simulink model "r_controller_system_integrated"  (R2025b)
settings: Solver=ode5  StartTime=0.0  StopTime=0.1  FixedStep=1e-05  MaxStep=1e-06  RelTol=1e-3
values from neighbouring files (symbols this model uses):
  params = Simulink.Parameter(params_data)    [r_controller_calc_params.m]
undefined symbols (not defined in the file or in its folder): Amplitude, Channel, ControllerType, d, Frequency, Ki_value, Kp_value, Phase, SignalType, StepTime
libraries: slpidlib x6, simulink x1
settings Model: Creator=PME406_01  LastModifiedBy=PME406_01
settings DebuggingCC: MergeDetectMultiDrivingBlocksExec=none
settings ModelReferenceCC: PropagateSignalLabelsOutOfModel=off

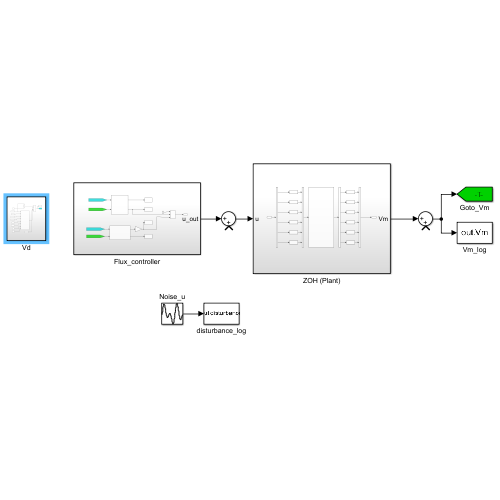
[thumbnail: Simulink's stored preview of the top-level diagram]
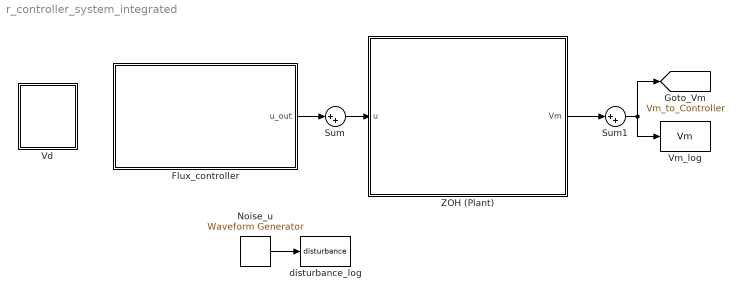
== system r_controller_system_integrated ==
  Flux_controller : Subsystem
  Noise_u : simulink/Sources/Waveform Generator  OutMin=[]  OutMax=[]  OutDataTypeStr=double  SelectedSignal=5  Signals=sin(0.1,10*2*pi, 0) + sin(0.1, 100*2*pi, pi/2) +sin(0.1,1000*2*pi, pi/4)#square(0.1,1000*2*pi,0,50)+square(0.1,500*2*pi,0,50)+square(0.1,50*2*pi,0,50)#sin(0.1,100*2*pi, pi/4)+sin(0.1,3000*2*pi,0)#square(0.1,50*2*pi,0,50)#sin(0.3, 100*2*pi, 0)#sawtooth(0.15,100*2*pi, pi/2)+sin(0.3, 100*2*pi, 0)#  BlockNames=MultiportSwitch_6f71199b286f490#MultiportSwitch_dade89289388493#MultiportSwitch_cf8a6d85c6a04a6#MultiportSwitch_8069dea399c144f#MultiportSwitch_735d7398da51477#MultiportSwitch_ae675588fc81459#MultiportSwitch_89d8400a71a24e9  SampleTime=1e-5
  Sum : Sum  Inputs=|++
  Sum1 : Sum  Inputs=|++
  Vd : Subsystem
  Vm_log : ToWorkspace  VariableName=Vm  SampleTime=1e-5
      settings: Save2DSignal=2-D array (concatenate along first dimension)
  ZOH (Plant) : Subsystem
  disturbance_log : ToWorkspace  VariableName=disturbance  SampleTime=1e-5
      settings: Save2DSignal=2-D array (concatenate along first dimension)
  tag scope: Vm_to_Controller=global
  wires:
  Noise_u/1 -> disturbance_log/1
  Sum1/1 -> Vm_log/1, [Vm_to_Controller]
  Sum/1 -> ZOH (Plant)/1(u)
  ZOH (Plant)/1(Vm) -> Sum1/1
  Flux_controller/1(u_out) -> Sum/1

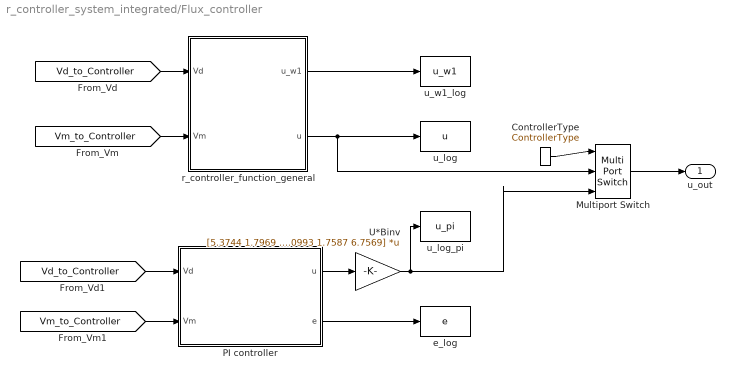
== system r_controller_system_integrated/Flux_controller ==
  ControllerType : Constant  Value=ControllerType
  Multiport Switch : MultiPortSwitch  Inputs=2  SaturateOnIntegerOverflow=off  InputSameDT=off
  PI controller : Subsystem
  U*Binv : Gain  Gain=[5.3744 1.7969 1.7574 2.2456 2.2738 2.0311;1.5722 5.8626 2.1621 3.1898 3.2303 2.3567;1.7622 2.0686 5.9804 1.8643 2.1053 2.1404;1.9445 3.4221 1.8713 6.8989 3.6309 2.3796;2.0590 3.2035 2.0193 3.4407 6.4464 2.0016;1.5291 2.0809 1.7335 2.0993 1.7587 6.7569]  Multiplication=Matrix(K*u)
  e_log : ToWorkspace  VariableName=e  SampleTime=-1
      settings: Save2DSignal=2-D array (concatenate along first dimension)
  r_controller_function_general : Subsystem
  u_log : ToWorkspace  VariableName=u  SampleTime=1e-5
      settings: Save2DSignal=2-D array (concatenate along first dimension)
  u_log_pi : ToWorkspace  VariableName=u_pi  SampleTime=-1
      settings: Save2DSignal=2-D array (concatenate along first dimension)
  u_w1_log : ToWorkspace  VariableName=u_w1  SampleTime=1e-5
      settings: Save2DSignal=2-D array (concatenate along first dimension)
  u_out : Outport
  wires:
  [Vd_to_Controller] -> r_controller_function_general/1(Vd)
  PI controller/1(u) -> U*Binv/1
  [Vd_to_Controller] -> PI controller/1(Vd)
  U*Binv/1 -> u_log_pi/1, Multiport Switch/3
  ControllerType/1 -> Multiport Switch/1
  [Vm_to_Controller] -> PI controller/2(Vm)
  r_controller_function_general/1(u_w1) -> u_w1_log/1
  r_controller_function_general/2(u) -> u_log/1, Multiport Switch/2
  [Vm_to_Controller] -> r_controller_function_general/2(Vm)
  PI controller/2(e) -> e_log/1
  Multiport Switch/1 -> u_out/1

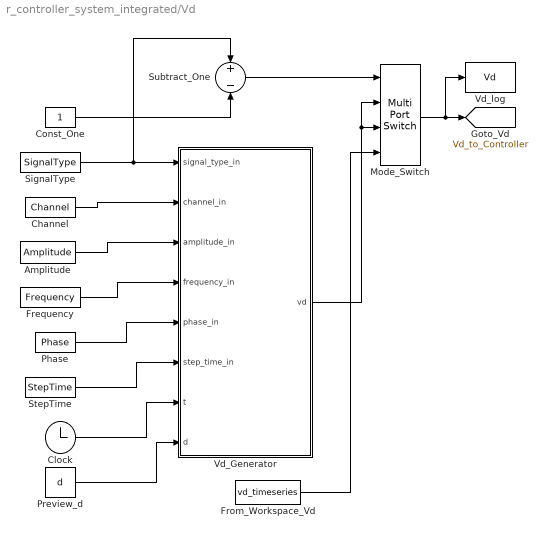
== system r_controller_system_integrated/Vd ==
  Amplitude : Constant  Value=Amplitude
  Channel : Constant  Value=Channel
  Clock : Clock
  Const_One : Constant
  Frequency : Constant  Value=Frequency
  From_Workspace_Vd : FromWorkspace  VariableName=vd_timeseries  SampleTime=1e-5  OutputAfterFinalValue=Holding final value
  Mode_Switch : MultiPortSwitch  DataPortOrder=Zero-based contiguous  zeroidx=on  SaturateOnIntegerOverflow=off  InputSameDT=off
  Phase : Constant  Value=Phase
  Preview_d : Constant  Value=d
  SignalType : Constant  Value=SignalType
  StepTime : Constant  Value=StepTime
  Subtract_One : Sum  Inputs=+-
  Vd_Generator : MATLAB Function  TreatAsAtomicUnit=on
  Vd_log : ToWorkspace  VariableName=Vd  SampleTime=1e-5
      settings: Save2DSignal=2-D array (concatenate along first dimension)
  tag scope: Vd_to_Controller=global
  wires:
  From_Workspace_Vd/1 -> Mode_Switch/4
  Vd_Generator/1(vd) -> Mode_Switch/3, Mode_Switch/2
  Preview_d/1 -> Vd_Generator/8(d)
  Clock/1 -> Vd_Generator/7(t)
  Frequency/1 -> Vd_Generator/4(frequency_in)
  StepTime/1 -> Vd_Generator/6(step_time_in)
  Channel/1 -> Vd_Generator/2(channel_in)
  Phase/1 -> Vd_Generator/5(phase_in)
  Amplitude/1 -> Vd_Generator/3(amplitude_in)
  Subtract_One/1 -> Mode_Switch/1
  SignalType/1 -> Vd_Generator/1(signal_type_in), Subtract_One/1
  Const_One/1 -> Subtract_One/2
  Mode_Switch/1 -> Vd_log/1, [Vd_to_Controller]

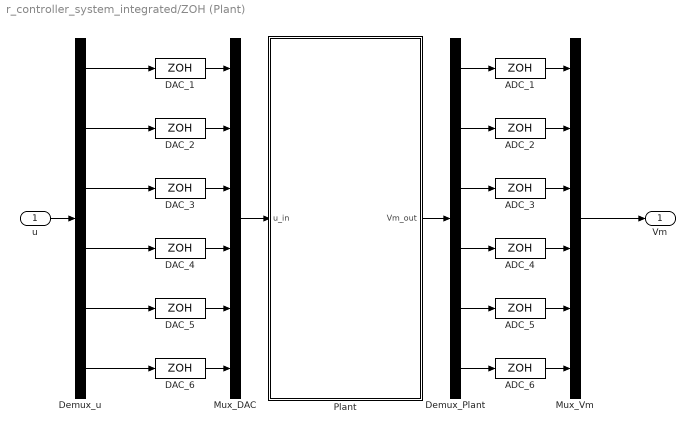
== system r_controller_system_integrated/ZOH (Plant) ==
  u : Inport
  ADC_{1..6} (6 alike) : ZeroOrderHold  SampleTime=1e-05
  DAC_{1..6} (6 alike) : ZeroOrderHold  SampleTime=1e-05
  Demux_Plant : Demux  Outputs=6
  Demux_u : Demux  Outputs=6
  Mux_DAC : Mux  Inputs=6
  Mux_Vm : Mux  Inputs=6
  Plant : Subsystem
  Vm : Outport
  wires:
  Demux_Plant/3 -> ADC_3/1
  DAC_2/1 -> Mux_DAC/2
  Demux_u/1 -> DAC_1/1
  Demux_u/6 -> DAC_6/1
  ADC_4/1 -> Mux_Vm/4
  DAC_3/1 -> Mux_DAC/3
  Mux_Vm/1 -> Vm/1
  Demux_Plant/2 -> ADC_2/1
  ADC_6/1 -> Mux_Vm/6
  Demux_Plant/1 -> ADC_1/1
  ADC_2/1 -> Mux_Vm/2
  Demux_u/5 -> DAC_5/1
  Plant/1(Vm_out) -> Demux_Plant/1
  Mux_DAC/1 -> Plant/1(u_in)
  DAC_1/1 -> Mux_DAC/1
  ADC_1/1 -> Mux_Vm/1
  Demux_u/4 -> DAC_4/1
  Demux_u/3 -> DAC_3/1
  Demux_Plant/6 -> ADC_6/1
  Demux_Plant/4 -> ADC_4/1
  ADC_3/1 -> Mux_Vm/3
  Demux_Plant/5 -> ADC_5/1
  DAC_4/1 -> Mux_DAC/4
  ADC_5/1 -> Mux_Vm/5
  DAC_5/1 -> Mux_DAC/5
  DAC_6/1 -> Mux_DAC/6
  Demux_u/2 -> DAC_2/1
  u/1 -> Demux_u/1

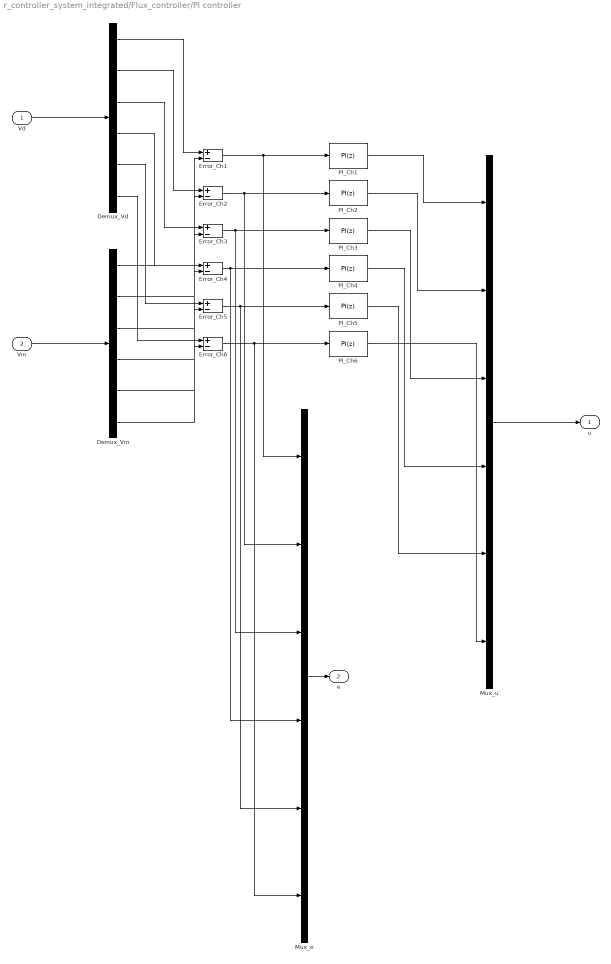
== system r_controller_system_integrated/Flux_controller/PI controller ==
  Vd : Inport
  Vm : Inport  Port=2
  Demux_Vd : Demux  Outputs=6
  Demux_Vm : Demux  Outputs=6
  Error_Ch{1..6} (6 alike) : Sum  Inputs=+-
  Mux_e : Mux  Inputs=6
  Mux_u : Mux  Inputs=6
  PI_Ch{1..2,4..6} (5 alike) : slpidlib/PID Controller  Controller=PI  Form=Parallel  TimeDomain=Discrete-time  UseExternalTs=off  SampleTime=1e-5  IntegratorMethod=Trapezoidal  FilterMethod=Forward Euler  ControllerParametersSource=internal  P=Kp_value  I=Ki_value  UseKiTs=off  D=0  UseExternalDerivativeSource=off  N=100  UseFilter=on  TunerSelectOption=Transfer Function Based (PID Tuner App)  InitialConditionSource=internal  InitialConditionForIntegrator=0  InitialConditionForFilter=0  DifferentiatorICPrevScaledInput=0  ExternalReset=none  TrackingMode=off  Kt=1  LimitOutput=off  SatLimitsSource=internal  UpperSaturationLimit=10  LowerSaturationLimit=-10  LinearizeAsGain=off  AntiWindupMode=back-calculation  Kb=1  LimitIntegrator=off  UpperIntegratorSaturationLimit=inf  LowerIntegratorSaturationLimit=-inf  POutMin=[]  POutMax=[]  IOutMin=[]  IOutMax=[]  DOutMin=[]  DOutMax=[]  NOutMin=[]  NOutMax=[]  SumOutMin=[]  SumOutMax=[]  SaturationOutMin=[]  SaturationOutMax=[]  PParamMin=[]  PParamMax=[]  IParamMin=[]  IParamMax=[]  DParamMin=[]  DParamMax=[]  NParamMin=[]  NParamMax=[]  KbParamMin=[]  KbParamMax=[]  KtParamMin=[]  KtParamMax=[]  KbOutMin=[]  KbOutMax=[]  KtOutMin=[]  KtOutMax=[]  IntegratorOutMin=[]  IntegratorOutMax=[]  FilterOutMin=[]  FilterOutMax=[]  SumI1OutMin=[]  SumI1OutMax=[]  SumI2OutMin=[]  SumI2OutMax=[]  SumI3OutMin=[]  SumI3OutMax=[]  SumI4OutMin=[]  SumI4OutMax=[]  SumDOutMin=[]  SumDOutMax=[]  DifferentiatorOutMin=[]  DifferentiatorOutMax=[]  FilterDiffOutCoefMin=[]  FilterDiffOutCoefMax=[]  ReciprocalOutMin=[]  ReciprocalOutMax=[]  SumDenOutMin=[]  SumDenOutMax=[]  SumNumOutMin=[]  SumNumOutMax=[]  DivideOutMin=[]  DivideOutMax=[]  UdiffTsProdOutMin=[]  UdiffTsProdOutMax=[]  NTsProdOutMin=[]  NTsProdOutMax=[]  UintegralTsProdOutMin=[]  UintegralTsProdOutMax=[]  UngainTsProdOutMin=[]  UngainTsProdOutMax=[]  ClampingZeroOutDataTypeStr=Inherit: Inherit via back propagation  ClampingZeroOutMin=[]  ClampingZeroOutMax=[]  FilterDenConstantOutDataTypeStr=Inherit: Inherit via back propagation  FilterDenConstantOutMin=[]  FilterDenConstantOutMax=[]  PCopyOutDataTypeStr=Inherit: Inherit via back propagation  PCopyOutMin=[]  PCopyOutMax=[]  NCopyOutDataTypeStr=Inherit: Inherit via back propagation  NCopyOutMin=[]  NCopyOutMax=[]  IntegratorContinuousStateAttributes=''  IntegratorStateMustResolveToSignalObject=off  IntegratorRTWStateStorageClass=Auto  FilterContinuousStateAttributes=''  FilterStateMustResolveToSignalObject=off  FilterRTWStateStorageClass=Auto  ParallelPVariant=InternalParameters  IdealPVariant=Disabled  IVariant=InternalParameters  DVariant=Disabled  IntegratorVariant=Discrete  SatVariant=Disabled  AWVariant=Passthrough  PCopyVariant=Disabled  TRVariant=Disabled  FdbkBlocksVariant=Forward  IdealPFdbkVariant=Disabled  SatFdbkVariant=Disabled  DerivativeFilterVariant=Disabled  NVariant=Disabled  NCopyVariant=Disabled_SignalSpec  FilterICVariant=Disabled  IntegratorICVariant=InternalICs  ExternalResetVariant=Disabled  TRSumVariant=Passthrough  SumFdbkVariant=Disabled  SumVariant=Sum_PI  TsampFilterVariant=InternalTs  TsampNgainVariant=Passthrough  TsampIntegralVariant=Disabled_SignalSpec  ExternalSaturationOutDataTypeStr=Inherit: Same as second input  DerivativeSourceVariant=Disabled  PreIntVariant=InternalPreInt
      settings: LibrarySourceBlock=simulink/Discrete/Discrete PID Controller
  PI_Ch3 : slpidlib/PID Controller  Controller=PI  Form=Parallel  TimeDomain=Discrete-time  UseExternalTs=off  SampleTime=1e-5  IntegratorMethod=Trapezoidal  FilterMethod=Forward Euler  ControllerParametersSource=internal  P=Kp_value  I=Ki_value  UseKiTs=off  D=0  UseExternalDerivativeSource=off  N=100  UseFilter=on  TunerSelectOption=Transfer Function Based (PID Tuner App)  InitialConditionSource=internal  InitialConditionForIntegrator=0  InitialConditionForFilter=0  DifferentiatorICPrevScaledInput=0  ExternalReset=none  TrackingMode=off  Kt=1  LimitOutput=off  SatLimitsSource=internal  UpperSaturationLimit=10  LowerSaturationLimit=-10  LinearizeAsGain=off  AntiWindupMode=back-calculation  Kb=1  LimitIntegrator=off  UpperIntegratorSaturationLimit=15  LowerIntegratorSaturationLimit=-15  POutMin=[]  POutMax=[]  IOutMin=[]  IOutMax=[]  DOutMin=[]  DOutMax=[]  NOutMin=[]  NOutMax=[]  SumOutMin=[]  SumOutMax=[]  SaturationOutMin=[]  SaturationOutMax=[]  PParamMin=[]  PParamMax=[]  IParamMin=[]  IParamMax=[]  DParamMin=[]  DParamMax=[]  NParamMin=[]  NParamMax=[]  KbParamMin=[]  KbParamMax=[]  KtParamMin=[]  KtParamMax=[]  KbOutMin=[]  KbOutMax=[]  KtOutMin=[]  KtOutMax=[]  IntegratorOutMin=[]  IntegratorOutMax=[]  FilterOutMin=[]  FilterOutMax=[]  SumI1OutMin=[]  SumI1OutMax=[]  SumI2OutMin=[]  SumI2OutMax=[]  SumI3OutMin=[]  SumI3OutMax=[]  SumI4OutMin=[]  SumI4OutMax=[]  SumDOutMin=[]  SumDOutMax=[]  DifferentiatorOutMin=[]  DifferentiatorOutMax=[]  FilterDiffOutCoefMin=[]  FilterDiffOutCoefMax=[]  ReciprocalOutMin=[]  ReciprocalOutMax=[]  SumDenOutMin=[]  SumDenOutMax=[]  SumNumOutMin=[]  SumNumOutMax=[]  DivideOutMin=[]  DivideOutMax=[]  UdiffTsProdOutMin=[]  UdiffTsProdOutMax=[]  NTsProdOutMin=[]  NTsProdOutMax=[]  UintegralTsProdOutMin=[]  UintegralTsProdOutMax=[]  UngainTsProdOutMin=[]  UngainTsProdOutMax=[]  ClampingZeroOutDataTypeStr=Inherit: Inherit via back propagation  ClampingZeroOutMin=[]  ClampingZeroOutMax=[]  FilterDenConstantOutDataTypeStr=Inherit: Inherit via back propagation  FilterDenConstantOutMin=[]  FilterDenConstantOutMax=[]  PCopyOutDataTypeStr=Inherit: Inherit via back propagation  PCopyOutMin=[]  PCopyOutMax=[]  NCopyOutDataTypeStr=Inherit: Inherit via back propagation  NCopyOutMin=[]  NCopyOutMax=[]  IntegratorContinuousStateAttributes=''  IntegratorStateMustResolveToSignalObject=off  IntegratorRTWStateStorageClass=Auto  FilterContinuousStateAttributes=''  FilterStateMustResolveToSignalObject=off  FilterRTWStateStorageClass=Auto  ParallelPVariant=InternalParameters  IdealPVariant=Disabled  IVariant=InternalParameters  DVariant=Disabled  IntegratorVariant=Discrete  SatVariant=Disabled  AWVariant=Passthrough  PCopyVariant=Disabled  TRVariant=Disabled  FdbkBlocksVariant=Forward  IdealPFdbkVariant=Disabled  SatFdbkVariant=Disabled  DerivativeFilterVariant=Disabled  NVariant=Disabled  NCopyVariant=Disabled_SignalSpec  FilterICVariant=Disabled  IntegratorICVariant=InternalICs  ExternalResetVariant=Disabled  TRSumVariant=Passthrough  SumFdbkVariant=Disabled  SumVariant=Sum_PI  TsampFilterVariant=InternalTs  TsampNgainVariant=Passthrough  TsampIntegralVariant=Disabled_SignalSpec  ExternalSaturationOutDataTypeStr=Inherit: Same as second input  DerivativeSourceVariant=Disabled  PreIntVariant=InternalPreInt
      settings: LibrarySourceBlock=simulink/Discrete/Discrete PID Controller
  u : Outport
  e : Outport  Port=2
  wires:
  Vd/1 -> Demux_Vd/1
  Vm/1 -> Demux_Vm/1
  Error_Ch5/1 -> PI_Ch5/1, Mux_e/5
  Demux_Vm/2 -> Error_Ch2/2
  Mux_u/1 -> u/1
  PI_Ch1/1 -> Mux_u/1
  PI_Ch4/1 -> Mux_u/4
  Error_Ch1/1 -> PI_Ch1/1, Mux_e/1
  Error_Ch3/1 -> PI_Ch3/1, Mux_e/3
  PI_Ch3/1 -> Mux_u/3
  Error_Ch6/1 -> PI_Ch6/1, Mux_e/6
  Error_Ch2/1 -> PI_Ch2/1, Mux_e/2
  Demux_Vm/5 -> Error_Ch5/2
  Demux_Vm/1 -> Error_Ch1/2
  Demux_Vd/2 -> Error_Ch2/1
  Demux_Vd/1 -> Error_Ch1/1
  PI_Ch2/1 -> Mux_u/2
  Demux_Vm/4 -> Error_Ch4/2
  Mux_e/1 -> e/1
  Demux_Vd/3 -> Error_Ch3/1
  Demux_Vd/6 -> Error_Ch6/1
  Error_Ch4/1 -> PI_Ch4/1, Mux_e/4
  Demux_Vd/5 -> Error_Ch5/1
  PI_Ch6/1 -> Mux_u/6
  PI_Ch5/1 -> Mux_u/5
  Demux_Vm/6 -> Error_Ch6/2
  Demux_Vm/3 -> Error_Ch3/2
  Demux_Vd/4 -> Error_Ch4/1

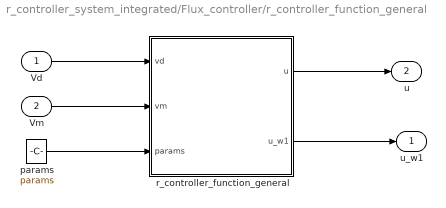
== system r_controller_system_integrated/Flux_controller/r_controller_function_general ==
  Vd : Inport
  Vm : Inport  Port=2
  params : Constant  Value=params  OutDataTypeStr=Bus: ParamsBus
  r_controller_function_general : MATLAB Function  TreatAsAtomicUnit=on
  u_w1 : Outport
  u : Outport  Port=2
  wires:
  r_controller_function_general/2(u_w1) -> u_w1/1
  Vm/1 -> r_controller_function_general/2(vm)
  Vd/1 -> r_controller_function_general/1(vd)
  r_controller_function_general/1(u) -> u/1
  params/1 -> r_controller_function_general/3(params)

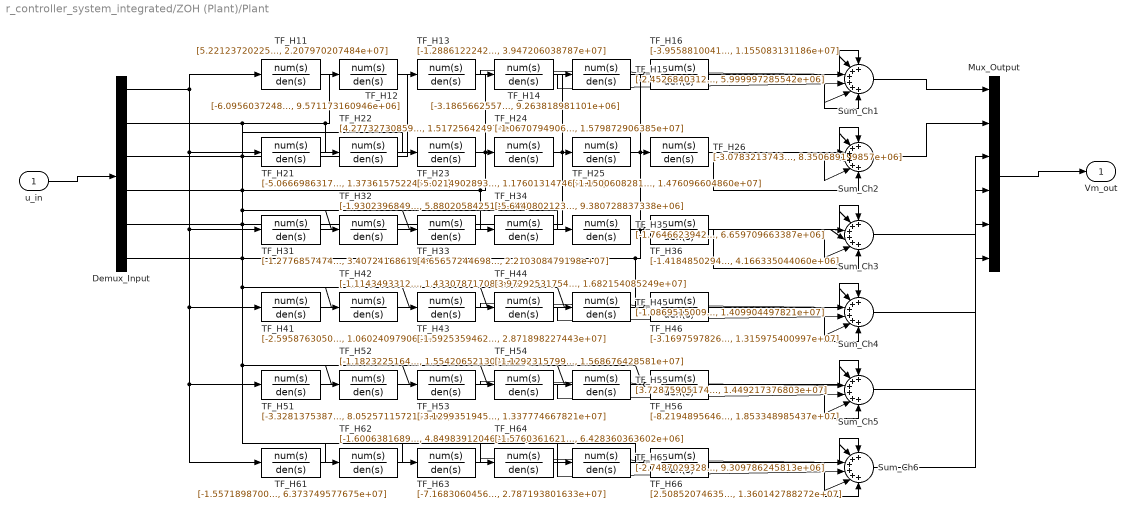
== system r_controller_system_integrated/ZOH (Plant)/Plant ==
  u_in : Inport
  Demux_Input : Demux  Outputs=6
  Mux_Output : Mux  Inputs=6
  Sum_Ch{1..6} (6 alike) : Sum  Inputs=++++++
  TF_H11 : TransferFcn  Numerator=[5.221237202258e+06]  Denominator=[1, 1.125476429798e+04, 2.207970207484e+07]
  TF_H12 : TransferFcn  Numerator=[-6.095603724823e+04]  Denominator=[1, 1.615096196557e+03, 9.571173160946e+06]
  TF_H13 : TransferFcn  Numerator=[-1.288612224236e+06]  Denominator=[1, 1.231137597589e+04, 3.947206038787e+07]
  TF_H14 : TransferFcn  Numerator=[-3.186566255776e+05]  Denominator=[1, 7.765927137710e+03, 9.263818981101e+06]
  TF_H15 : TransferFcn  Numerator=[-2.452684031253e+05]  Denominator=[1, 5.746401647961e+03, 5.999997285542e+06]
  TF_H16 : TransferFcn  Numerator=[-3.955881004140e+05]  Denominator=[1, 3.580306515557e+03, 1.155083131186e+07]
  TF_H21 : TransferFcn  Numerator=[-5.066698631790e+04]  Denominator=[1, 1.108261849372e+03, 1.373615752245e+07]
  TF_H22 : TransferFcn  Numerator=[4.277327308593e+06]  Denominator=[1, 1.003268373777e+04, 1.517256424974e+07]
  TF_H23 : TransferFcn  Numerator=[-5.021490289304e+05]  Denominator=[1, 8.810895080316e+03, 1.176013147465e+07]
  TF_H24 : TransferFcn  Numerator=[-1.067079490600e+06]  Denominator=[1, 1.135112820448e+04, 1.579872906385e+07]
  TF_H25 : TransferFcn  Numerator=[-1.150060828107e+06]  Denominator=[1, 1.065992916636e+04, 1.476096604860e+07]
  TF_H26 : TransferFcn  Numerator=[-3.078321374306e+05]  Denominator=[1, 6.847783968129e+03, 8.350689199857e+06]
  TF_H31 : TransferFcn  Numerator=[-1.277685747428e+06]  Denominator=[1, 1.368269686933e+04, 3.407241686199e+07]
  TF_H32 : TransferFcn  Numerator=[-1.930239684968e+05]  Denominator=[1, 4.560870597302e+03, 5.880205842512e+06]
  TF_H33 : TransferFcn  Numerator=[4.656572446985e+06]  Denominator=[1, 9.513164457161e+03, 2.210308479198e+07]
  TF_H34 : TransferFcn  Numerator=[-5.644080212304e+04]  Denominator=[1, 1.954878812118e+03, 9.380728837338e+06]
  TF_H35 : TransferFcn  Numerator=[-1.764662394212e+05]  Denominator=[1, 5.122349981324e+03, 6.659709663387e+06]
  TF_H36 : TransferFcn  Numerator=[-1.418485029440e+05]  Denominator=[1, 1.438504147902e+03, 4.166335044060e+06]
  TF_H41 : TransferFcn  Numerator=[-2.595876305066e+05]  Denominator=[1, 7.070165651413e+03, 1.060240979066e+07]
  TF_H42 : TransferFcn  Numerator=[-1.114349331223e+06]  Denominator=[1, 9.846928206402e+03, 1.433078717084e+07]
  TF_H43 : TransferFcn  Numerator=[-1.592535946272e+05]  Denominator=[1, 2.790294019501e+03, 2.871898227443e+07]
  TF_H44 : TransferFcn  Numerator=[3.972925317547e+06]  Denominator=[1, 1.159715140811e+04, 1.682154085249e+07]
  TF_H45 : TransferFcn  Numerator=[-1.086951500933e+06]  Denominator=[1, 1.075231371220e+04, 1.409904497821e+07]
  TF_H46 : TransferFcn  Numerator=[-3.169759782656e+05]  Denominator=[1, 8.067558736035e+03, 1.315975400997e+07]
  TF_H51 : TransferFcn  Numerator=[-3.328137538766e+05]  Denominator=[1, 7.227274813518e+03, 8.052571157216e+06]
  TF_H52 : TransferFcn  Numerator=[-1.182322516481e+06]  Denominator=[1, 1.030784744910e+04, 1.554206521303e+07]
  TF_H53 : TransferFcn  Numerator=[-3.129935194599e+05]  Denominator=[1, 7.870328655037e+03, 1.337774667821e+07]
  TF_H54 : TransferFcn  Numerator=[-1.129231579925e+06]  Denominator=[1, 1.104821595243e+04, 1.568676428581e+07]
  TF_H55 : TransferFcn  Numerator=[3.728759051745e+06]  Denominator=[1, 1.050075182774e+04, 1.449217376803e+07]
  TF_H56 : TransferFcn  Numerator=[-8.219489564647e+04]  Denominator=[1, 1.407969854523e+03, 1.853348985437e+07]
  TF_H61 : TransferFcn  Numerator=[-1.557189870041e+06]  Denominator=[1, 2.234640585923e+04, 6.373749577675e+07]
  TF_H62 : TransferFcn  Numerator=[-1.600638168987e+05]  Denominator=[1, 3.864055922471e+03, 4.849839120469e+06]
  TF_H63 : TransferFcn  Numerator=[-7.168306045699e+05]  Denominator=[1, 9.251556589809e+03, 2.787193801633e+07]
  TF_H64 : TransferFcn  Numerator=[-1.576036162155e+05]  Denominator=[1, 4.743270970318e+03, 6.428360363602e+06]
  TF_H65 : TransferFcn  Numerator=[-2.748702932822e+04]  Denominator=[1, 4.876033357949e+02, 9.309786245813e+06]
  TF_H66 : TransferFcn  Numerator=[2.508520746356e+06]  Denominator=[1, 5.985310903650e+03, 1.360142788272e+07]
  Vm_out : Outport
  wires:
  Sum_Ch3/1 -> Mux_Output/3
  TF_H36/1 -> Sum_Ch3/6
  TF_H16/1 -> Sum_Ch1/6
  TF_H63/1 -> Sum_Ch6/3
  Demux_Input/2 -> TF_H52/1, TF_H62/1, TF_H42/1, TF_H32/1, TF_H12/1, TF_H22/1
  TF_H23/1 -> Sum_Ch2/3
  TF_H31/1 -> Sum_Ch3/1
  Sum_Ch1/1 -> Mux_Output/1
  TF_H51/1 -> Sum_Ch5/1
  TF_H12/1 -> Sum_Ch1/2
  TF_H61/1 -> Sum_Ch6/1
  TF_H22/1 -> Sum_Ch2/2
  Demux_Input/4 -> TF_H54/1, TF_H64/1, TF_H44/1, TF_H14/1, TF_H24/1, TF_H34/1
  TF_H14/1 -> Sum_Ch1/4
  TF_H62/1 -> Sum_Ch6/2
  TF_H25/1 -> Sum_Ch2/5
  Sum_Ch4/1 -> Mux_Output/4
  TF_H41/1 -> Sum_Ch4/1
  TF_H45/1 -> Sum_Ch4/5
  Sum_Ch6/1 -> Mux_Output/6
  TF_H54/1 -> Sum_Ch5/4
  TF_H64/1 -> Sum_Ch6/4
  TF_H55/1 -> Sum_Ch5/5
  Demux_Input/6 -> TF_H56/1, TF_H66/1, TF_H16/1, TF_H26/1, TF_H36/1, TF_H46/1
  TF_H42/1 -> Sum_Ch4/2
  TF_H13/1 -> Sum_Ch1/3
  TF_H26/1 -> Sum_Ch2/6
  TF_H21/1 -> Sum_Ch2/1
  Demux_Input/5 -> TF_H55/1, TF_H65/1, TF_H45/1, TF_H15/1, TF_H25/1, TF_H35/1
  Sum_Ch2/1 -> Mux_Output/2
  u_in/1 -> Demux_Input/1
  TF_H44/1 -> Sum_Ch4/4
  TF_H24/1 -> Sum_Ch2/4
  TF_H66/1 -> Sum_Ch6/6
  TF_H43/1 -> Sum_Ch4/3
  TF_H33/1 -> Sum_Ch3/3
  TF_H52/1 -> Sum_Ch5/2
  Demux_Input/3 -> TF_H53/1, TF_H63/1, TF_H43/1, TF_H33/1, TF_H13/1, TF_H23/1
  TF_H15/1 -> Sum_Ch1/5
  TF_H56/1 -> Sum_Ch5/6
  TF_H32/1 -> Sum_Ch3/2
  TF_H34/1 -> Sum_Ch3/4
  TF_H53/1 -> Sum_Ch5/3
  Demux_Input/1 -> TF_H51/1, TF_H61/1, TF_H41/1, TF_H31/1, TF_H21/1, TF_H11/1
  TF_H11/1 -> Sum_Ch1/1
  TF_H35/1 -> Sum_Ch3/5
  Mux_Output/1 -> Vm_out/1
  Sum_Ch5/1 -> Mux_Output/5
  TF_H65/1 -> Sum_Ch6/5
  TF_H46/1 -> Sum_Ch4/6

== matlab function r_controller_system_integrated/Flux_controller/r_controller_function_general/r_controller_function_general ==
  settings: updateMethod=DISCRETE  sampleTime=1e-5
  data: vd input size=6; u output size=6; vm input size=6; u_w1 output size=6; params input
function [u, u_w1] = fcn(vd, vm, params)
    [u, u_w1] = r_controller_function_general(vd, vm, params);
end

== matlab function r_controller_system_integrated/Vd/Vd_Generator ==
  settings: updateMethod=DISCRETE  sampleTime=1e-5
  data: signal_type_in input; channel_in input; amplitude_in input; frequency_in input; phase_in input; step_time_in input; t input; vd output size=6; d input
function vd = fcn(signal_type_in, channel_in, amplitude_in, frequency_in, phase_in, step_time_in, t, d)
% Vd Generator - Sine Wave and Step modes
% Mode 3 (External) is handled by From Workspace block + Switch

    Ts = 1e-5;
    t_future = t + Ts * d;

    vd = zeros(6, 1);

    channel = round(channel_in);
    if channel < 1 || channel > 6
        channel = 1;
    end

    if signal_type_in == 1
        % Sine Wave
        vd(channel) = amplitude_in * sin(2*pi*frequency_in*t_future + deg2rad(phase_in));
    else
        % Step
        if t_future >= step_time_in
            vd(channel) = amplitude_in;
        else
            vd(channel) = 0;
        end
    end
end
